simulink model "SolarPanelTracker"  (R2024b)
settings: Solver=FixedStepDiscrete  StartTime=0.0  StopTime=10.0  FixedStep=1e-3  RelTol=1e-3
settings Model: Creator=MOHAMED  LastModifiedBy=MOHAMED
settings OptimizationCC: DefaultParameterBehavior=Inlined  UseDivisionForNetSlopeComputation=on  GainParamInheritBuiltInType=on  UseFloatMulNetSlope=on  InlineInvariantSignals=on  PassReuseOutputArgsAs=Individual arguments  ZeroExternalMemoryAtStartup=off  ZeroInternalMemoryAtStartup=off  NoFixptDivByZeroProtection=on  EfficientFloat2IntCast=on  LifeSpan=1  OptimizeBlockOrder=speed  DifferentSizesBufferReuse=on  EfficientTunableParamExpr=on
settings DebuggingCC: ParameterTunabilityLossMsg=error
settings HardwareCC: ProdLongLongMode=on
settings SFSimCC: MATLABDynamicMemAlloc=off
settings RTWCC: Description=Embedded Coder  SystemTargetFile=ert.tlc  TemplateMakefile=ert_default_tmf
settings CodeAppCC: ForceParamTrailComments=on  IgnoreCustomStorageClasses=off  OperatorAnnotations=on  SimulinkDataObjDesc=on  SFDataObjDesc=on  CustomSymbolStrGlobalVar=rt$N$M  CustomSymbolStrType=$N$M  CustomSymbolStrFcn=$N$M$F  CustomSymbolStrMacro=$N$M  InsertBlockDesc=on
settings ERTTargetCC: TargetLangStandard=C99 (ISO)  GenerateSampleERTMain=on  IncludeMdlTerminateFcn=off  CombineSignalStateStructs=on  SupportAbsoluteTime=off  SupportComplex=off  SupportNonInlinedSFcns=on  ERTCustomFileTemplate=example_file_process.tlc  ERTFilePackagingFormat=CompactWithDataFile

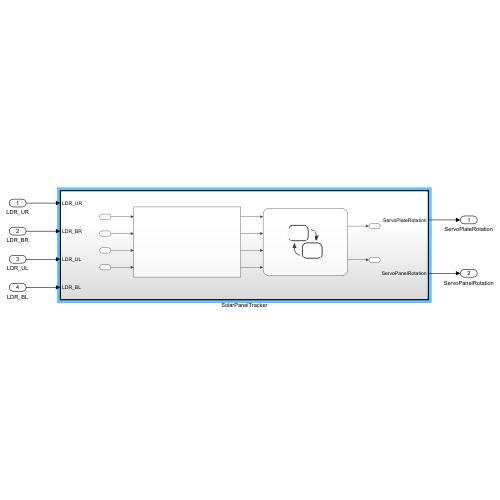
[thumbnail: Simulink's stored preview of the top-level diagram]
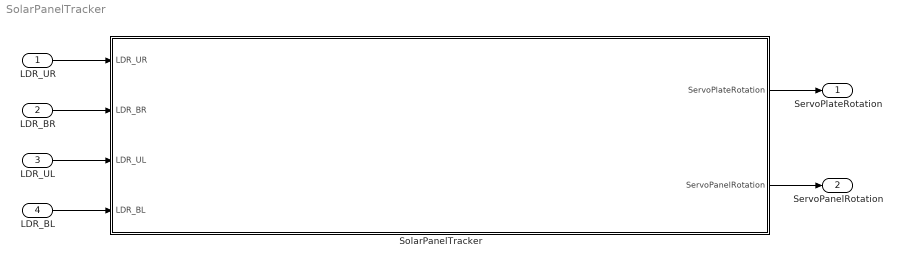
== system SolarPanelTracker ==
  LDR_UR : Inport
  LDR_BR : Inport  Port=2
  LDR_UL : Inport  Port=3
  LDR_BL : Inport  Port=4
  SolarPanelTracker : Subsystem  TreatAsAtomicUnit=on
  ServoPlateRotation : Outport
  ServoPanelRotation : Outport  Port=2
  wires:
  LDR_UR/1 -> SolarPanelTracker/1(LDR_UR)
  SolarPanelTracker/1(ServoPlateRotation) -> ServoPlateRotation/1
  LDR_BL/1 -> SolarPanelTracker/4(LDR_BL)
  LDR_UL/1 -> SolarPanelTracker/3(LDR_UL)
  LDR_BR/1 -> SolarPanelTracker/2(LDR_BR)
  SolarPanelTracker/2(ServoPanelRotation) -> ServoPanelRotation/1

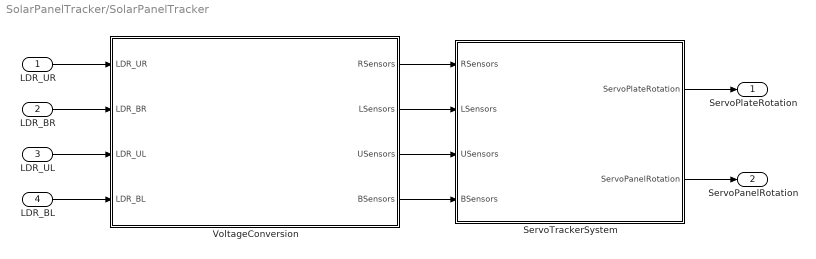
== system SolarPanelTracker/SolarPanelTracker ==
  LDR_UR : Inport
  LDR_BR : Inport  Port=2
  LDR_UL : Inport  Port=3
  LDR_BL : Inport  Port=4
  ServoTrackerSystem : Stateflow chart  TreatAsAtomicUnit=on
  VoltageConversion : Subsystem  TreatAsAtomicUnit=on
  ServoPlateRotation : Outport
  ServoPanelRotation : Outport  Port=2
  wires:
  LDR_UR/1 -> VoltageConversion/1(LDR_UR)
  LDR_BR/1 -> VoltageConversion/2(LDR_BR)
  LDR_UL/1 -> VoltageConversion/3(LDR_UL)
  LDR_BL/1 -> VoltageConversion/4(LDR_BL)
  VoltageConversion/1(RSensors) -> ServoTrackerSystem/1(RSensors)
  VoltageConversion/2(LSensors) -> ServoTrackerSystem/2(LSensors)
  VoltageConversion/4(BSensors) -> ServoTrackerSystem/4(BSensors)
  VoltageConversion/3(USensors) -> ServoTrackerSystem/3(USensors)
  ServoTrackerSystem/1(ServoPlateRotation) -> ServoPlateRotation/1
  ServoTrackerSystem/2(ServoPanelRotation) -> ServoPanelRotation/1

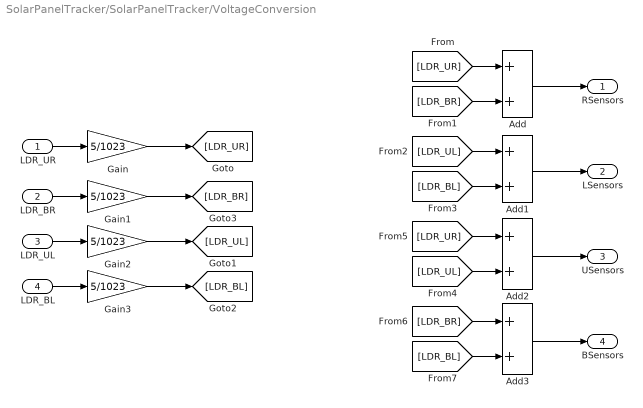
== system SolarPanelTracker/SolarPanelTracker/VoltageConversion ==
  LDR_UR : Inport
  LDR_BR : Inport  Port=2
  LDR_UL : Inport  Port=3
  LDR_BL : Inport  Port=4
  Add{,1..3} (4 alike) : Sum
  Gain{,1..3} (4 alike) : Gain  Gain=5/1023
  RSensors : Outport
  LSensors : Outport  Port=2
  USensors : Outport  Port=3
  BSensors : Outport  Port=4
  wires:
  LDR_BR/1 -> Gain1/1
  LDR_UL/1 -> Gain2/1
  LDR_UR/1 -> Gain/1
  LDR_BL/1 -> Gain3/1
  Gain/1 -> [LDR_UR]
  Gain2/1 -> [LDR_UL]
  Gain3/1 -> [LDR_BL]
  Gain1/1 -> [LDR_BR]
  [LDR_UR] -> Add/1
  [LDR_BR] -> Add/2
  [LDR_UL] -> Add1/1
  [LDR_BL] -> Add1/2
  [LDR_UL] -> Add2/2
  [LDR_UR] -> Add2/1
  [LDR_BR] -> Add3/1
  [LDR_BL] -> Add3/2
  Add3/1 -> BSensors/1
  Add2/1 -> USensors/1
  Add1/1 -> LSensors/1
  Add/1 -> RSensors/1

== stateflow chart SolarPanelTracker/ServoTrackerSystem ==
  state PanelServo [parallel]
    settings: executionOrder=1
    (default) -> (junction 8)
    PanelServo -> (junction 8)
    (junction 8) -> (junction 13) [order 1] : [abs(RSensors - LSensors) <= 0.5]
    (junction 8) -> (junction 17) [order 2]
    (junction 13) -> (junction 15) : {ServoPanelRotation = 0;}
    (junction 17) -> (junction 19) [order 1] : [RSensors > LSensors]
    (junction 17) -> (junction 20) [order 2] : {ServoPanelRotation = LSensors/2 * 255/5 * ServoStepAngle;}
    (junction 19) -> (junction 23) : {ServoPanelRotation = RSensors/2 * 255/5 * ServoStepAngle;}
    (junction 23) -> (junction 20)
    (junction 15) -> (junction 23)
    (junction 20) -> (junction 27)
  state PlateServo [parallel]
    settings: executionOrder=2
    (default) -> (junction 68)
    PlateServo -> (junction 68)
    (junction 68) -> (junction 52) [order 1] : [abs(USensors - BSensors) <= 0.5]
    (junction 68) -> (junction 71) [order 2]
    (junction 52) -> (junction 67) : {ServoPlateRotation = 0;}
    (junction 71) -> (junction 64) [order 1] : [USensors > BSensors]
    (junction 71) -> (junction 72) [order 2] : {ServoPlateRotation = BSensors/2 * 255/5 * ServoStepAngle;}
    (junction 64) -> (junction 63) : {ServoPlateRotation = USensors/2 * 255/5 * ServoStepAngle;}
    (junction 63) -> (junction 72)
    (junction 67) -> (junction 63)
    (junction 72) -> (junction 61)
  data: RSensors input; LSensors input; USensors input; BSensors input; ServoPlateRotation output; ServoPanelRotation output; ServoStepAngle local double =180/255
